simulink model "Mostar"  (Simulink 10.1)
settings: Solver=ode45  StartTime=0  StopTime=136  FixedStep=0.01  RelTol=0.001  EnableMultiTasking=on
libraries: fmu_me_lib x1
settings Model: Creator=Tin Rabuzin  LastModifiedBy=meagh
settings DataIOCC: LimitDataPoints=on  OutputSaveName=simout  OutputOption=SpecifiedOutputTimes  OutputTimes=[0:0.5:136]
settings OptimizationCC: ExpressionDepthLimit=2147483647
settings DebuggingCC: SolverPrmCheckMsg=warning  StateNameClashWarn=warning
settings GRTTargetCC: CombineOutputUpdateFcns=on  GRTInterface=off

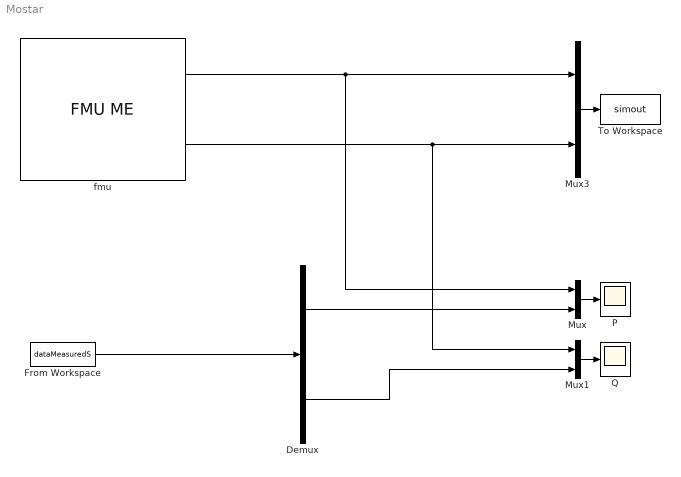
== system Mostar ==
  Demux : Demux  Outputs=2
  From Workspace : FromWorkspace  VariableName=dataMeasuredS
  Mux : Mux  Inputs=2
  Mux1 : Mux  Inputs=2
  Mux3 : Mux  Inputs=2
  P : Scope
  Q : Scope
  To Workspace : ToWorkspace  VariableName=simout  SaveFormat=Structure With Time  SampleTime=0.5
  fmu : fmu_me_lib/FMU ME  Description=Simulates an FMU for Model Exchange 1.0 or Model Exchange 2.0.  dummy=0
  wires:
  From Workspace/1 -> Demux/1
  Mux3/1 -> To Workspace/1
  fmu/1 -> Mux/1, Mux3/1
  Demux/1 -> Mux/2
  fmu/2 -> Mux1/1, Mux3/2
  Demux/2 -> Mux1/2
  Mux/1 -> P/1
  Mux1/1 -> Q/1
